simulink model "wss_noise"  (R2024a)
settings: Solver=VariableStepAuto  StartTime=0.0  StopTime=10  RelTol=1e-3
libraries: simulink x1
settings Model: Creator=Columbia  LastModifiedBy=benjaminlevin
settings RTWCC: GPUComputeCapability=3.5

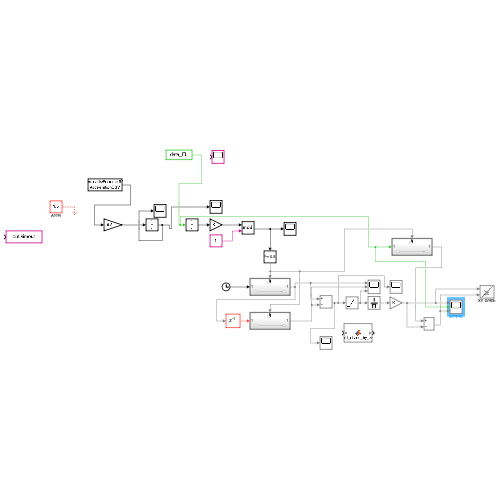
[thumbnail: Simulink's stored preview of the top-level diagram]
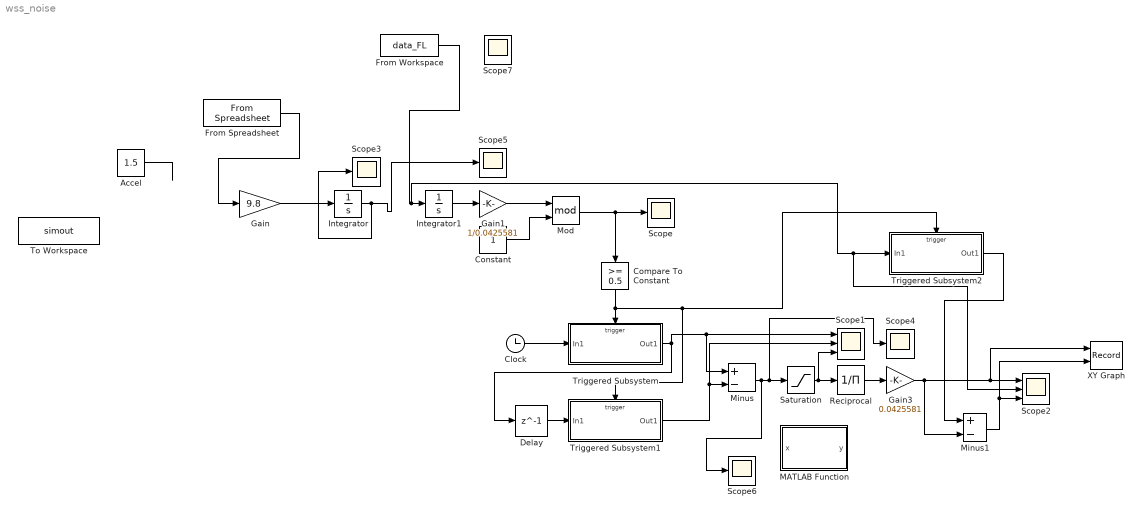
== system wss_noise ==
  Accel : Constant  Value=1.5  SampleTime=0.001
  Clock : Clock
  Compare To Constant : simulink/Logic and Bit Operations/Compare To Constant  relop=>=  const=0.5  OutDataTypeStr=boolean
  Constant : Constant
  Delay : Delay  DelayLength=1
  From Workspace : FromWorkspace  VariableName=data_FL  SampleTime=0.002
  From Spreadsheet : FromSpreadsheet  FileName=/Users/benjaminlevin/Downloads/Formula SAE/AccelerationCSV.xlsx  SheetName=AccelerationCSV  Range=A1:B76416
  Gain : Gain  Gain=9.8
  Gain1 : Gain  Gain=1/0.0425581
  Gain3 : Gain  Gain=0.0425581
  Integrator : Integrator
  Integrator1 : Integrator
  MATLAB Function : MATLAB Function  TreatAsAtomicUnit=on
  Minus : Sum  Inputs=+-
  Minus1 : Sum  Inputs=+-
  Mod : Math  Operator=mod
  Reciprocal : Product  Inputs=/
  Saturation : Saturate  UpperLimit=inf  LowerLimit=1e-6
  Scope{,3..7} (6 alike) : Scope
  Scope1 : Scope  NumInputPorts=3
  Scope2 : Scope  NumInputPorts=3
  To Workspace : ToWorkspace  VariableName=simout  SaveFormat=Timeseries  SampleTime=-1
  Triggered Subsystem : Subsystem  TreatAsAtomicUnit=on
  Triggered Subsystem1 : Subsystem  TreatAsAtomicUnit=on
  Triggered Subsystem2 : Subsystem  TreatAsAtomicUnit=on
  XY Graph : Record  FileSettingsInternal="{\"entries\":[{\"content\":{\"excelSettings\":{\"content\":{},\"type\":\"Streamout.ExcelSettings\"}},\"type\":\"Streamout.FileSettingStorage\",\"uuid\":\"\"}],\"packageUris\":[\"http:\\/\\/schema.mathworks.com\\/mf0\\/streamout_blocks\\/R2020a\"],\"version\":\"1.0\"}"  Layout=[1 1]  SignalsInternal="{\"entries\":[{\"content\":{\"signals\":[{\"content\":{\"blockPath\":[],\"dimensions\":[1],\"domain\":\"\",\"lineColor\":\"#ff13a6\",\"lineWidth\":2,\"port\":1,\"sid\":[\"\"],\"signalID\":1,\"signalName\":\"Gain3\"},\"type\":\"RecordBlkView.Signal\",\"uuid\":\"\"},{\"content\":{\"blockPath\":[],\"dimensions\":[1,1],\"domain\":\"\",\"lineColor\":\"#fe330a\",\"lineWidth\":2,\"port\":2,\"sid\":[\"\"],\"signalID\":2,\"signalName\":\"Minus1\"},\"type\":\"RecordBlkView.Signal\",\"uuid\":\"\"}]},\"type\":\"RecordBlkView.InputSignals\",\"uuid\":\"\"}],\"packageUris\":[\"http:\\/\\/schema.mathworks.com\\/mf0\\/streamout_blocks\\/R2020a\"],\"version\":\"1.0\"}"  VisualizationBindings="{\"xyplotplugin\":{\"info\":[{\"series\":[],\"subplotID\":1}]}}"  CompatibilityTag=XY
  wires:
  Accel/1 -> ?
  Gain/1 -> Integrator/1
  Integrator/1 -> Scope3/1, Scope5/1
  Integrator1/1 -> Gain1/1
  Gain1/1 -> Mod/1
  Mod/1 -> Scope/1, Compare To Constant/1
  Clock/1 -> Triggered Subsystem/1(In1)
  Triggered Subsystem/1(Out1) -> Scope1/1, Minus/1, Delay/1
  Constant/1 -> Mod/2
  Compare To Constant/1 -> Triggered Subsystem2/Trigger, Triggered Subsystem1/Trigger, Triggered Subsystem/Trigger
  Delay/1 -> Triggered Subsystem1/1(In1)
  Triggered Subsystem1/1(Out1) -> Minus/2, Scope1/2
  Minus/1 -> Scope6/1, Saturation/1, Scope4/1
  Gain3/1 -> Minus1/2, Scope2/1, XY Graph/1
  Reciprocal/1 -> Gain3/1
  Minus1/1 -> Scope2/3, XY Graph/2
  Triggered Subsystem2/1(Out1) -> Minus1/1
  Saturation/1 -> Scope1/3, Reciprocal/1
  From Spreadsheet/1 -> Gain/1
  From Workspace/1 -> Scope2/2, Triggered Subsystem2/1(In1), Integrator1/1

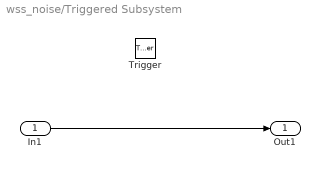
== system wss_noise/Triggered Subsystem ==
  In1 : Inport
  Trigger : TriggerPort  TriggerType=falling  VariantControl=(inherit)
  Out1 : Outport
  wires:
  In1/1 -> Out1/1

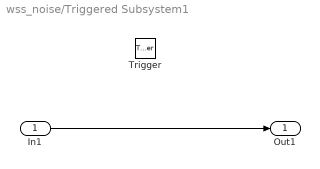
== system wss_noise/Triggered Subsystem1 ==
  In1 : Inport
  Trigger : TriggerPort  TriggerType=falling  VariantControl=(inherit)
  Out1 : Outport
  wires:
  In1/1 -> Out1/1

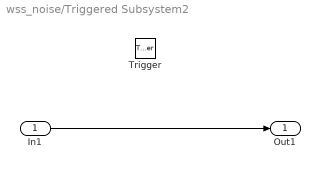
== system wss_noise/Triggered Subsystem2 ==
  In1 : Inport
  Trigger : TriggerPort  TriggerType=falling  VariantControl=(inherit)
  Out1 : Outport
  wires:
  In1/1 -> Out1/1

== matlab function wss_noise/MATLAB Function ==
  data: x input; y output
function y = avoid_divide_by_zero(x)
    threshold = 1e-6; % Small nonzero threshold
    if abs(x) < threshold
        y = sign(x) * threshold; % Preserve sign and avoid zero
    else
        y = x;
    end
end
